simulink model "Trajectory_Design"  (Simulink 9.1)
settings: Solver=VariableStepAuto  StartTime=0.0  StopTime=10.0  RelTol=1e-3
settings Model: Creator=78253  LastModifiedBy=syy
settings DataIOCC: SaveFormat=Dataset  ReturnWorkspaceOutputs=on
settings OptimizationCC: LifeSpan=auto
settings DebuggingCC: UnderspecifiedInitializationDetection=Simplified  MergeDetectMultiDrivingBlocksExec=error  SFUnexpectedBacktrackingDiag=error  SFNoUnconditionalDefaultTransitionDiag=error  SFExecutionAtInitializationDiag=warning
settings HardwareCC: ProdBitPerPointer=64  ProdBitPerSizeT=64  ProdBitPerPtrDiffT=64  ProdLargestAtomicFloat=Float  ProdIntDivRoundTo=Zero  ProdEndianess=LittleEndian  ProdWordSize=64  ProdHWDeviceType=Intel->x86-64 (Windows64)
settings ModelReferenceCC: PropagateSignalLabelsOutOfModel=on
settings SFSimCC: SimUseLocalCustomCode=on
settings RTWCC: RTWUseLocalCustomCode=on
settings CodeAppCC: StateflowObjectComments=off
settings GRTTargetCC: TargetLangStandard=C99 (ISO)  CombineOutputUpdateFcns=on  GRTInterface=off
settings ConfigComp: CovMetricSettings=dwe  CovHtmlReporting=off  CovSaveCumulativeToWorkspaceVar=off  CovSaveSingleToWorkspaceVar=off  CovExternalEMLEnable=on

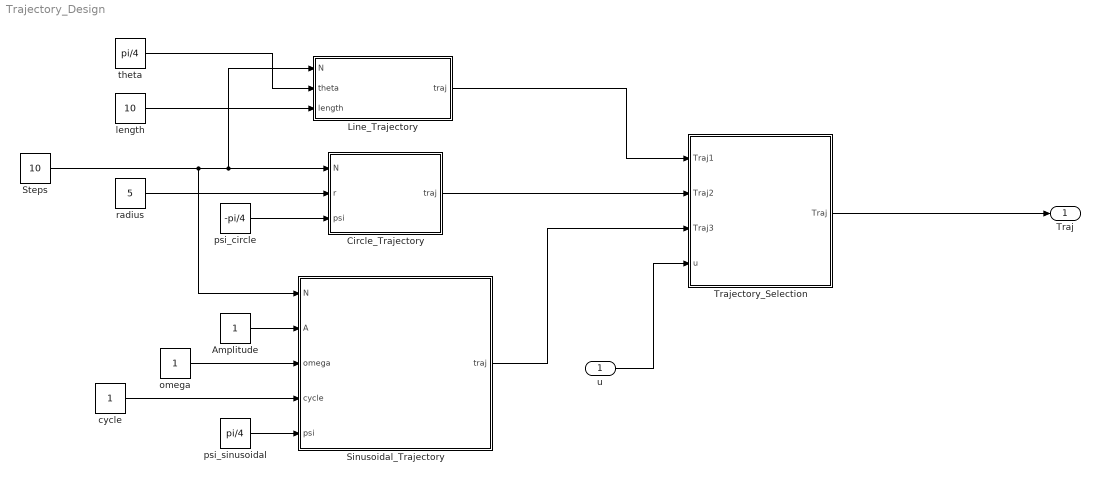
== system Trajectory_Design ==
  u : Inport
  Amplitude : Constant
  Circle_Trajectory : MATLAB Function  TreatAsAtomicUnit=on
  Line_Trajectory : MATLAB Function  TreatAsAtomicUnit=on
  Sinusoidal_Trajectory : MATLAB Function  TreatAsAtomicUnit=on
  Steps : Constant  Value=10
  Trajectory_Selection : MATLAB Function  TreatAsAtomicUnit=on
  cycle : Constant
  length : Constant  Value=10
  omega : Constant
  psi_circle : Constant  Value=-pi/4
  psi_sinusoidal : Constant  Value=pi/4
  radius : Constant  Value=5
  theta : Constant  Value=pi/4
  Traj : Outport
  wires:
  u/1 -> Trajectory_Selection/4(u)
  Trajectory_Selection/1(Traj) -> Traj/1
  Steps/1 -> Sinusoidal_Trajectory/1(N), Circle_Trajectory/1(N), Line_Trajectory/1(N)
  Line_Trajectory/1(traj) -> Trajectory_Selection/1(Traj1)
  theta/1 -> Line_Trajectory/2(theta)
  length/1 -> Line_Trajectory/3(length)
  Circle_Trajectory/1(traj) -> Trajectory_Selection/2(Traj2)
  radius/1 -> Circle_Trajectory/2(r)
  Sinusoidal_Trajectory/1(traj) -> Trajectory_Selection/3(Traj3)
  psi_circle/1 -> Circle_Trajectory/3(psi)
  psi_sinusoidal/1 -> Sinusoidal_Trajectory/5(psi)
  Amplitude/1 -> Sinusoidal_Trajectory/2(A)
  omega/1 -> Sinusoidal_Trajectory/3(omega)
  cycle/1 -> Sinusoidal_Trajectory/4(cycle)

== matlab function Line_Trajectory ==
  data: N input double; traj output double; theta input double; length input double
function traj = Line_Traj(N, theta, length)
% N+1 is the number of sampled points along the trajectory,
% including the start and the end.
% Thus, from the start point to the end point, there are N steps.

% theta is the dip angle by the x-axis, thus the slope k = tan(theta).
% theta is radian instead of degree.

% length is the length of the line trajectory.

length_x = length * cos(theta);
length_y = length * sin(theta);

px = zeros(N+1, 1); py = zeros(N+1, 1);
for i = 1 : N+1
    px(i) = length_x/N * (i-1);
    py(i) = length_y/N * (i-1);
end

traj = [px, py];

== matlab function Trajectory_Selection ==
  data: Traj1 input double; Traj2 input double; Traj3 input double; u input double; Traj output double
function Traj = Traj_Sel( Traj1, Traj2, Traj3, u)
% Trajectory Selection
% Traj divided by 10 is for scaling
if u == 1
    Traj = Traj1/10;
elseif u == 2
    Traj = Traj2/10;
elseif u == 3
    Traj = Traj3/10;
else
    Traj = Traj1/10;
end

== matlab function Circle_Trajectory ==
  data: N input double; traj output double; r input double; psi input double
function traj = Cir_Traj(N, r, psi)
% First we only care about the specific circle that satisfies
% x^2 + (y-r)^2 = r^2, where r is the radius of the circle.
% And in the polar coordinate system, it is:
% ρ = 2*r*sin(θ), where θ is between 0 and π.

% From the start point to the end point, there are N steps.
% Thus we divide π into N segments, that is, for the i th point sampled in
% the trajectory, its polar coordinate (ρi,θi) = (2*r*sin(θi), θi),
% where θi = (π/N)*(i-1).
% Finally, change the polar coordinate back to the Cartesian (xi, yi).

% Then, if the circle is rotated around the origin by ψ counterclockwise,
% we just do a coordinate transformation.

px = zeros(N+1, 1); py = zeros(N+1, 1);
for i = 1 : N+1
    theta_i = (pi/N) * (i-1);
    rou_i = 2 * r * sin(theta_i);
    px_t = rou_i * cos(theta_i);
    py_t = rou_i * sin(theta_i);
    % coordinate transformation when the circle is rotated by psi
    px(i) = px_t * cos(psi) - py_t * sin(psi);
    py(i) = px_t * sin(psi) + py_t * cos(psi);
end

traj = [px, py];

== matlab function Sinusoidal_Trajectory ==
  data: N input double; traj output double; A input double; omega input double; cycle input double; psi input double
function traj = Sin_Traj(N, A, omega, cycle, psi)
% We always and only focus on the sinusoidal curve whose phase is 0.

% First we only care about the sinusoidal curve that expands along the
% x-axis, that is, y = A * sin(ω*t).
% cycle is how many cycles we're going along the sinusoidal trajectory.
% Thus, the distance we're going along on the component of the x-axis is:
% dis_on_x = (2π/ω) * cycle.

% From the start point to the end point, there are N steps.
% Thus we divide dis_on_x into N segments, that is, for the i th point
% sampled in the trajectory, (xi, yi) = (xi, A*sin(omega*xi)),
% where xi = (dis_on_x/N)*(i-1).

% Then, if the circle is rotated around the origin by ψ counterclockwise,
% we just do a coordinate transformation.

dis_on_x = (2*pi/omega) * cycle;

px = zeros(N+1, 1); py = zeros(N+1, 1);
for i = 1 : N+1
    px_t = (dis_on_x/N) * (i-1);
    py_t = A * sin(omega * px_t);
    % coordinate transformation when the circle is rotated by psi
    px(i) = px_t * cos(psi) - py_t * sin(psi);
    py(i) = px_t * sin(psi) + py_t * cos(psi);
end

traj = N;
